simulink model "rev0_PEM"  (R2024a)
settings: Solver=VariableStepAuto  StartTime=0.0  StopTime=10.0  RelTol=1e-3
libraries: spsParallelRLCBranchLib x12, spsDiodeLib x4, spsIdealSwitchLib x4, spsControlledVoltageSourceLib x2, spsDCVoltageSourceLib x1
settings Model: Creator=ADMIN  LastModifiedBy=ADMIN

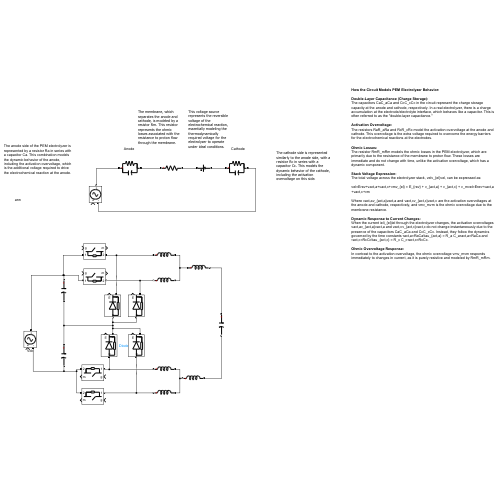
[thumbnail: Simulink's stored preview of the top-level diagram]
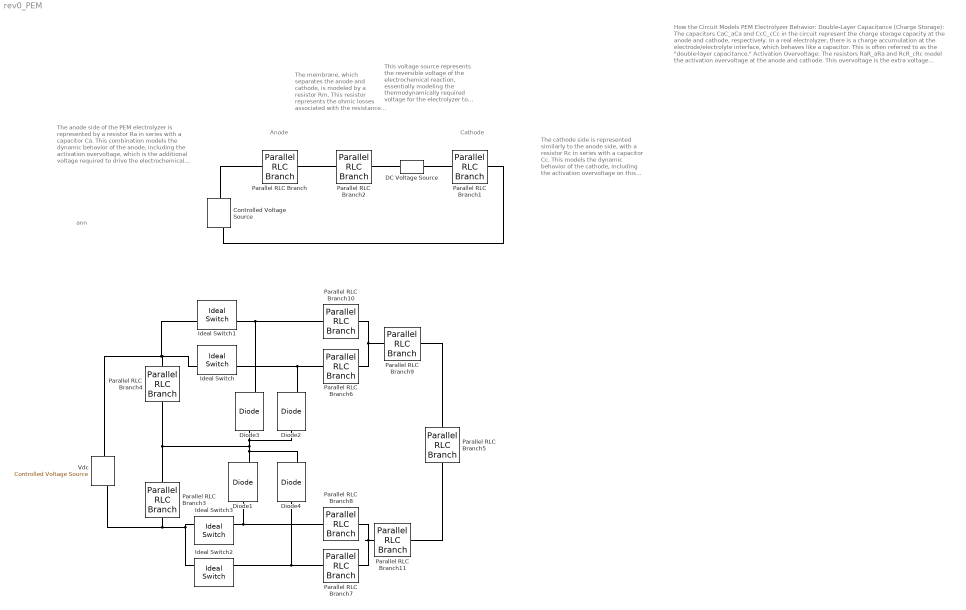
== system rev0_PEM ==
  note: How the Circuit Models PEM Electrolyzer Behavior:
      | Double-Layer Capacitance (Charge Storage):
      | The capacitors CaC_aCa​ and CcC_cCc​ in the circuit represent the charge storage capacity at the anode and cathode, respectively. In a real electrolyzer, there is a charge accumulation at the electrode/electrolyte interface, which behaves like a capacitor. This is often referred to as the "double-layer capacitance."
      | Activation Overvoltage:
      | The resistors RaR_aRa​ and RcR_cRc​ model the activation overvoltage at the anode and cathode. This overvoltage is the extra voltage required to overcome the energy barriers for the electrochemical reactions at the electrodes.
      | Ohmic Losses:
      | The resistor RmR_mRm​ models the ohmic losses in the PEM electrolyzer, which are primarily due to the resistance of the membrane to proton flow. These losses are immediate and do not change with time, unlike the activation overvoltage, which has a dynamic component.
      | Stack Voltage Expression:
      | The total voltage across the electrolyzer stack, velv_{el}vel​, can be expressed as:
      | vel=Erev+vact,a+vact,c+vmv_{el} = E_{rev} + v_{act,a} + v_{act,c} + v_mvel​=Erev​+vact,a​+vact,c​+vm​
      | Where vact,av_{act,a}vact,a​ and vact,cv_{act,c}vact,c​ are the activation overvoltages at the anode and cathode, respectively, and vmv_mvm​ is the ohmic overvoltage due to the membrane resistance.
      | Dynamic Response to Current Changes:
      | When the current ieli_{el}iel​ through the electrolyzer changes, the activation overvoltages vact,av_{act,a}vact,a​ and vact,cv_{act,c}vact,c​ do not change instantaneously due to the presence of the capacitors CaC_aCa​ and CcC_cCc​. Instead, they follow the dynamics governed by the time constants τact,a=RaCa\tau_{act,a} = R_a C_aτact,a​=Ra​Ca​ and τact,c=RcCc\tau_{act,c} = R_c C_cτact,c​=Rc​Cc​.
      | Ohmic Overvoltage Response:
      | In contrast to the activation overvoltage, the ohmic overvoltage vmv_mvm​ responds immediately to changes in current, as it is purely resistive and modeled by RmR_mRm​.
  note: This voltage source represents the reversible voltage of the electrochemical reaction, essentially modeling the thermodynamically required voltage for the electrolyzer to operate under ideal conditions.
  note: The cathode side is represented similarly to the anode side, with a resistor Rc​ in series with a capacitor Cc. This models the dynamic behavior of the cathode, including the activation overvoltage on this side.
  note: The membrane, which separates the anode and cathode, is modeled by a resistor Rm​. This resistor represents the ohmic losses associated with the resistance to proton flow through the membrane.
  note: ann
  note: The anode side of the PEM electrolyzer is represented by a resistor Ra​ in series with a capacitor Ca​. This combination models the dynamic behavior of the anode, including the activation overvoltage, which is the additional voltage required to drive the electrochemical reaction at the anode.
  note: Cathode
  note: Anode
  Controlled Voltage Source : spsControlledVoltageSourceLib/Controlled Voltage Source  Initialize=on  Source_Type=AC  Amplitude=0  Phase=0  Frequency=0  Measurements=None
  DC Voltage Source : spsDCVoltageSourceLib/DC Voltage Source  Amplitude=100  Measurements=None
  Diode{1..4} (4 alike) : spsDiodeLib/Diode  Ron=0.001  Lon=0  Vf=0.8  IC=0  UseSnubber=0  Rs=500  Cs=250e-9  Measurements=on
  Ideal Switch{,1..3} (4 alike) : spsIdealSwitchLib/Ideal Switch  Ron=0.001  Lon=0  IC=0  Rs=1e5  Cs=inf  Measurements=on
  Parallel RLC Branch : spsParallelRLCBranchLib/Parallel RLC Branch  LConnTagsString=a  RConnTagsString=__new0  BranchType=RC  Resistance=1  Inductance=1e-3  SetiL0=off  InitialCurrent=0  Capacitance=1e-6  Setx0=off  InitialVoltage=0  Measurements=None
  Parallel RLC Branch1 : spsParallelRLCBranchLib/Parallel RLC Branch  LConnTagsString=a  RConnTagsString=__new0  BranchType=RC  Resistance=1  Inductance=1e-3  SetiL0=off  InitialCurrent=0  Capacitance=1e-6  Setx0=off  InitialVoltage=0  Measurements=None
  Parallel RLC Branch{6..11} (6 alike) : spsParallelRLCBranchLib/Parallel RLC Branch  LConnTagsString=a  RConnTagsString=__new0  BranchType=L  Resistance=1  Inductance=1e-3  SetiL0=off  InitialCurrent=0  Capacitance=1e-6  Setx0=off  InitialVoltage=0  Measurements=None
  Parallel RLC Branch2 : spsParallelRLCBranchLib/Parallel RLC Branch  LConnTagsString=a  RConnTagsString=__new0  BranchType=R  Resistance=1  Inductance=1e-3  SetiL0=off  InitialCurrent=0  Capacitance=1e-6  Setx0=off  InitialVoltage=0  Measurements=None
  Parallel RLC Branch3 : spsParallelRLCBranchLib/Parallel RLC Branch  LConnTagsString=a  RConnTagsString=__new0  BranchType=C  Resistance=1  Inductance=1e-3  SetiL0=off  InitialCurrent=0  Capacitance=1e-6  Setx0=off  InitialVoltage=0  Measurements=None
  Parallel RLC Branch4 : spsParallelRLCBranchLib/Parallel RLC Branch  LConnTagsString=a  RConnTagsString=__new0  BranchType=C  Resistance=1  Inductance=1e-3  SetiL0=off  InitialCurrent=0  Capacitance=1e-6  Setx0=off  InitialVoltage=0  Measurements=None
  Parallel RLC Branch5 : spsParallelRLCBranchLib/Parallel RLC Branch  LConnTagsString=a  RConnTagsString=__new0  BranchType=C  Resistance=1  Inductance=1e-3  SetiL0=off  InitialCurrent=0  Capacitance=1e-6  Setx0=off  InitialVoltage=0  Measurements=None
  Vdc : spsControlledVoltageSourceLib/Controlled Voltage Source  Initialize=on  Source_Type=AC  Amplitude=0  Phase=0  Frequency=0  Measurements=None
  connections:
  Parallel RLC Branch/RConn1 -- Parallel RLC Branch2/LConn1
  Parallel RLC Branch1/RConn1 -- Controlled Voltage Source/LConn1
  DC Voltage Source/RConn1 -- Parallel RLC Branch2/RConn1
  Parallel RLC Branch1/LConn1 -- DC Voltage Source/LConn1
  Controlled Voltage Source/RConn1 -- Parallel RLC Branch/LConn1
  Diode2/LConn1 -- Diode4/RConn1 -- Diode1/RConn1 -- Parallel RLC Branch3/LConn1 -- Parallel RLC Branch4/RConn1 -- Diode3/LConn1
  Vdc/RConn1 -- Ideal Switch/LConn1 -- Parallel RLC Branch4/LConn1 -- Ideal Switch1/LConn1
  Ideal Switch3/RConn1 -- Vdc/LConn1 -- Parallel RLC Branch3/RConn1 -- Ideal Switch2/RConn1
  Parallel RLC Branch6/LConn1 -- Ideal Switch/RConn1 -- Diode2/RConn1
  Ideal Switch1/RConn1 -- Diode3/RConn1 -- Parallel RLC Branch10/LConn1
  Parallel RLC Branch6/RConn1 -- Parallel RLC Branch9/LConn1 -- Parallel RLC Branch10/RConn1
  Parallel RLC Branch9/RConn1 -- Parallel RLC Branch5/LConn1
  Parallel RLC Branch8/LConn1 -- Diode1/LConn1 -- Ideal Switch3/LConn1
  Parallel RLC Branch7/LConn1 -- Diode4/LConn1 -- Ideal Switch2/LConn1
  Parallel RLC Branch7/RConn1 -- Parallel RLC Branch11/LConn1 -- Parallel RLC Branch8/RConn1
  Parallel RLC Branch11/RConn1 -- Parallel RLC Branch5/RConn1
